simulink model "Sim1"  (R2023b)
settings: Solver=VariableStepAuto  StartTime=0.0  StopTime=10.0  RelTol=1e-3
model workspace (MAT data in the model file):
  g = 9.8
  l = 0.8
  m = 2
settings Model: Creator=surrlim  LastModifiedBy=surrlim

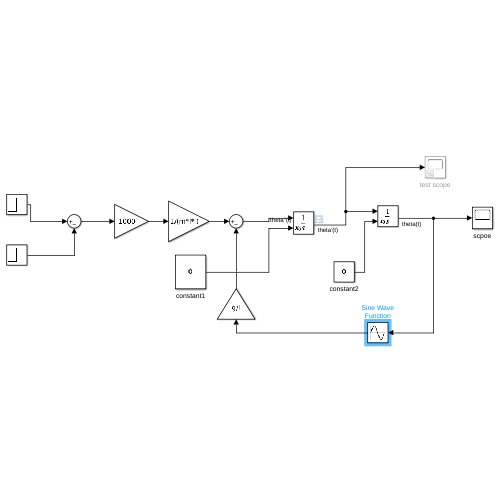
[thumbnail: Simulink's stored preview of the top-level diagram]
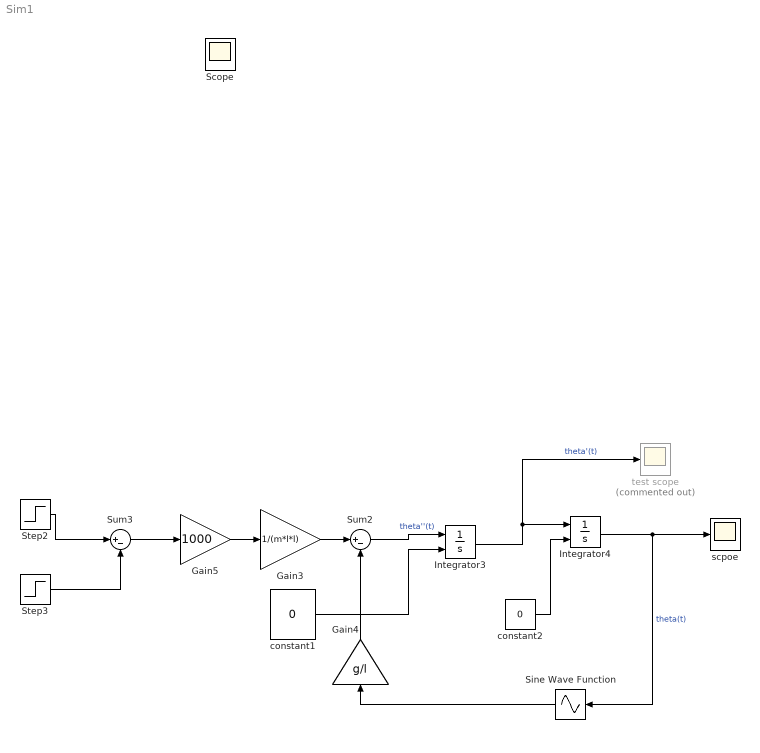
== system Sim1 ==
  Gain3 : Gain  Gain=1/(m*l*l)
  Gain4 : Gain  Gain=g/l
  Gain5 : Gain  Gain=1000
  Integrator3 : Integrator  InitialConditionSource=external  InitialCondition=1/(m*l*l)
  Integrator4 : Integrator  InitialConditionSource=external
  Sine Wave Function : Sin  TimeSource=Use external signal  Frequency=1/(2*pi)  SampleTime=0
  Step2 : Step  Time=0  SampleTime=0
  Step3 : Step  Time=0.001  SampleTime=0
  Sum2 : Sum  Inputs=|+-
  Sum3 : Sum  Inputs=|+-
  constant1 : Constant  Value=0
  constant2 : Constant  Value=0
  scpoe : Scope
  test scope : Scope  Commented=on
  Scope : Scope
  wires:
  Step2/1 -> Sum3/1
  Gain3/1 -> Sum2/1
  Sum2/1 -> Integrator3/1  "theta''(t)"
  Sine Wave Function/1 -> Gain4/1
  Gain4/1 -> Sum2/2
  Step3/1 -> Sum3/2
  Sum3/1 -> Gain5/1
  Integrator3/1 -> test scope/1, Integrator4/1  "theta'(t)"
  constant2/1 -> Integrator4/2
  Integrator4/1 -> Sine Wave Function/1, scpoe/1  "theta(t)"
  Gain5/1 -> Gain3/1
  constant1/1 -> Integrator3/2
